simulink library "rsd"  (Simulink 8.1)
settings: Solver=ode1  StartTime=0.0  StopTime=Inf  FixedStep=0.001  RelTol=1e-3
PostLoadFcn:
  | , if any(exist('dsrtsu_mdlpostloadfcn', 'file') == [2, 3, 6]), try dsrtsu_mdlpostloadfcn('Execute', bdroot); catch fprintf('Error in PostLoadFcn (dsrtsu_mdlpostloadfcn) for model "%s":\n %s\n', bdroot, lasterr); end, end,
undefined symbols (not defined in the file or in its folder): AACC_ACCDistVehSpd_kph, FALSE, KACC_ACCDistErrorGParam_num, KACC_ACCDistFFParam_num, KACC_ACCDistInitialIParam_num, KACC_ACCDistKdParam_num, KACC_ACCDistKiParam_num, KACC_ACCDistKpParam_num, KACC_ACCDistMaxIParam_num, KACC_ACCDistMinIParam_num, KACC_ACCDistResetIParam_num, MACC_DistPIDErrorG_num, MACC_DistPIDKp_num
libraries: hcu_lib x2
settings Model: DSRTSU_INTERNAL_RTI_VER=450  DSRTSU_INTERNAL_RTI_TYPE=rti1401  RTICANMMDATA=struct('GeneralSetupData',struct('modelroot','D:\ELN150201_TAIWAN\trunk\AdasDragon\software\sw_development\arch\app\acc','generalsettings',struct('filesettings',struct('destfolder',struct('Name','RTICANMM_FILES','Check',1),'buildfolder',struct('Name','.','Check',1),'AbsDestfolder',struct('Name','D:\ELN150201_TAIWAN\trunk\AdasDragon\software\sw_development\arch\app\acc\RTICANMM_FILES'),'AbsBuildfolder',struct('Name','D:\ELN150201_TAIWAN\trunk\AdasDragon\software\sw_development\arch\app\acc'))),'options',struct('addpaths',1,'rmpaths',1,'addtrcexclusion',logical(1),'cannavigator',struct('checkmonitoring',0),'show_usrtrc',0,'use_usrtrc',0),'advanced',struct('options',[1 1 1 1 1 1 1 1 1 1 1 1 1 1 1 1 1 1 1 1 1 1 1 1 1 1 1 1 1 1 1 1 1 1 1 1 1 1 1 1 1 1 1 1 1 1 1 1 1 1 1 1 1 1 1 1 1 1 1 1 1 1 1 1 1 1 1 1 1 1 1 1 1 1 1 1 1 1 1 1 1 1 1 1 1 1 1 1 1 1 1 1 1 1 1 1 1 1 1 1]),'MPSetup',{{}},'modelname','rsd','block','rsd'))  DSRTSU_INTERNAL_RTIFPGA=40  Creator=AT015555  LastModifiedBy=AT015555

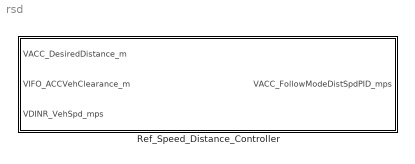
== system rsd ==
  Ref_Speed_Distance_Controller : Subsystem

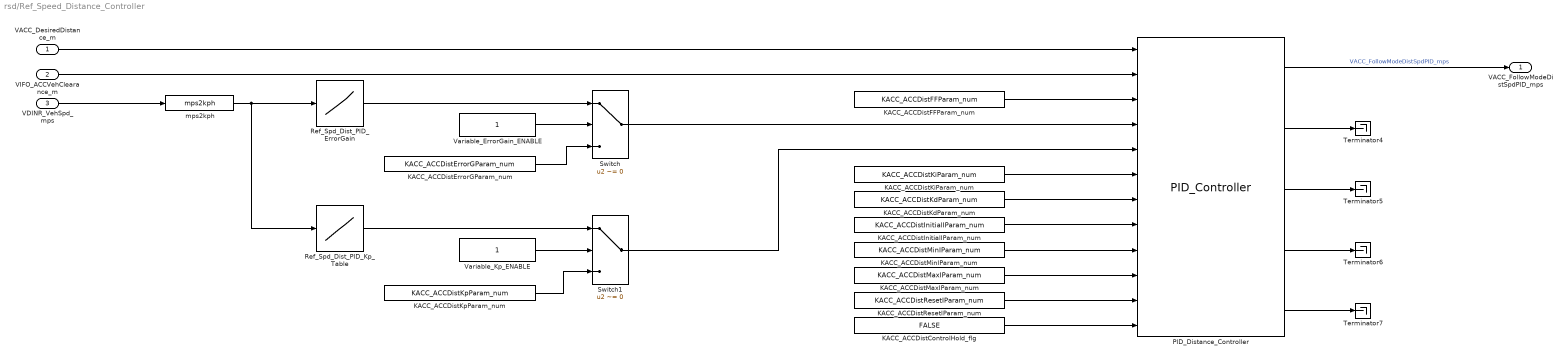
== system rsd/Ref_Speed_Distance_Controller ==
  VACC_DesiredDistance_m : Inport
  VIFO_ACCVehClearance_m : Inport  Port=2
  VDINR_VehSpd_mps : Inport  Port=3
  KACC_ACCDistControlHold_flg : Constant  Value=FALSE  OutDataTypeStr=boolean
  KACC_ACCDistErrorGParam_num : Constant  Value=KACC_ACCDistErrorGParam_num
  KACC_ACCDistFFParam_num : Constant  Value=KACC_ACCDistFFParam_num
  KACC_ACCDistInitialIParam_num : Constant  Value=KACC_ACCDistInitialIParam_num
  KACC_ACCDistKdParam_num : Constant  Value=KACC_ACCDistKdParam_num
  KACC_ACCDistKiParam_num : Constant  Value=KACC_ACCDistKiParam_num
  KACC_ACCDistKpParam_num : Constant  Value=KACC_ACCDistKpParam_num
  KACC_ACCDistMaxIParam_num : Constant  Value=KACC_ACCDistMaxIParam_num
  KACC_ACCDistMinIParam_num : Constant  Value=KACC_ACCDistMinIParam_num
  KACC_ACCDistResetIParam_num : Constant  Value=KACC_ACCDistResetIParam_num
  PID_Distance_Controller : hcu_lib/PID_Controller  SystemSampleTime=-1
  Ref_Spd_Dist_PID_ErrorGain : Lookup_n-D  NumberOfTableDimensions=1  BreakpointsForDimension1=AACC_ACCDistVehSpd_kph  Table=MACC_DistPIDErrorG_num  ExtrapMethod=Clip  UseLastTableValue=on  RndMeth=Simplest  InputSameDT=on
  Ref_Spd_Dist_PID_Kp_Table : Lookup_n-D  NumberOfTableDimensions=1  BreakpointsForDimension1=AACC_ACCDistVehSpd_kph  Table=MACC_DistPIDKp_num  ExtrapMethod=Clip  UseLastTableValue=on  RndMeth=Simplest  InputSameDT=on
  Switch : Switch  Criteria=u2 ~= 0
  Switch1 : Switch  Criteria=u2 ~= 0
  Terminator{4..7} (4 alike) : Terminator
  Variable_ErrorGain_ENABLE : Constant  OutDataTypeStr=boolean
  Variable_Kp_ENABLE : Constant  OutDataTypeStr=boolean
  mps2kph : hcu_lib/mps2kph
  VACC_FollowModeDistSpdPID_mps : Outport
  wires:
  VACC_DesiredDistance_m/1 -> PID_Distance_Controller/1
  PID_Distance_Controller/3 -> Terminator5/1
  Switch1/1 -> PID_Distance_Controller/5
  PID_Distance_Controller/2 -> Terminator4/1
  VIFO_ACCVehClearance_m/1 -> PID_Distance_Controller/2
  PID_Distance_Controller/4 -> Terminator6/1
  KACC_ACCDistMinIParam_num/1 -> PID_Distance_Controller/9
  PID_Distance_Controller/5 -> Terminator7/1
  KACC_ACCDistFFParam_num/1 -> PID_Distance_Controller/3
  KACC_ACCDistInitialIParam_num/1 -> PID_Distance_Controller/8
  KACC_ACCDistKiParam_num/1 -> PID_Distance_Controller/6
  PID_Distance_Controller/1 -> VACC_FollowModeDistSpdPID_mps/1  "VACC_FollowModeDistSpdPID_mps"
  KACC_ACCDistControlHold_flg/1 -> PID_Distance_Controller/12
  KACC_ACCDistMaxIParam_num/1 -> PID_Distance_Controller/10
  KACC_ACCDistResetIParam_num/1 -> PID_Distance_Controller/11
  KACC_ACCDistKdParam_num/1 -> PID_Distance_Controller/7
  Variable_ErrorGain_ENABLE/1 -> Switch/2
  Switch/1 -> PID_Distance_Controller/4
  KACC_ACCDistErrorGParam_num/1 -> Switch/3
  Ref_Spd_Dist_PID_ErrorGain/1 -> Switch/1
  VDINR_VehSpd_mps/1 -> mps2kph/1
  mps2kph/1 -> Ref_Spd_Dist_PID_Kp_Table/1, Ref_Spd_Dist_PID_ErrorGain/1
  Variable_Kp_ENABLE/1 -> Switch1/2
  KACC_ACCDistKpParam_num/1 -> Switch1/3
  Ref_Spd_Dist_PID_Kp_Table/1 -> Switch1/1
